simulink model "HW_InterleavedTotemBridgelessPFC_PR_V11_R2022a_AVE19"  (R2022a)
settings: Solver=FixedStepDiscrete  StartTime=0.0  StopTime=0.5  FixedStep=Ts_Power  RelTol=1e-3
InitFcn:
  | clc;
  | clear;
  | 
  | %%simulation paremeter
  | fsw = 130e3;%switch freq
  | Ts_Control = 1/fsw * 2;%control period
  | Ts_Power = 1 / fsw/128;%simulation step
  | Ts_Sample = 1 / fsw;%sample period
  | Tscon = Ts_Control;
  | %%system parameter
  | L = 250e-6;
  | L1 = L;
  | L2 = L;
  | C = 620e-6;
  | R = 75;
  | Uc_init = 390 ;%capacitor voltage init
  | v_ref = 390;
  | 
  | %%controller parameter
  | k_cp=-0.0235;
  | k_ci=-1.871e3;
  | 
  | k_vi = 1.7714;
  | k_vp = 0.0488;
undefined symbols (not defined in the file or in its folder): DiscIntNeverNeededParam
libraries: spsSeriesRLCBranchLib x3, slpidlib x2, spsCurrentMeasurementLib x2, spsVoltageMeasurementLib x2, spsACVoltageSourceLib x1, dsparch4 x1, spsPWMGenerator2LevelLib x1, spsStairGeneratorLib x1, spsTwoQuadrantDCDCConverterLib x1, spsUniversalBridgeLib x1, spspowerguiLib x1
settings Model: Creator=xg  LastModifiedBy=12586
settings SolverCC: AlgebraicLoopSolver=TrustRegion
settings DataIOCC: ReturnWorkspaceOutputs=off
settings DebuggingCC: ArithmeticOperatorsInVariantConditions=warning
settings SFSimCC: CustomCodeUndefinedFunction=UseInterfaceOnly

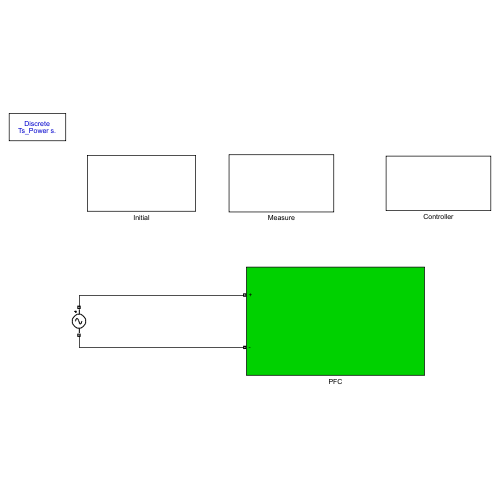
[thumbnail: Simulink's stored preview of the top-level diagram]
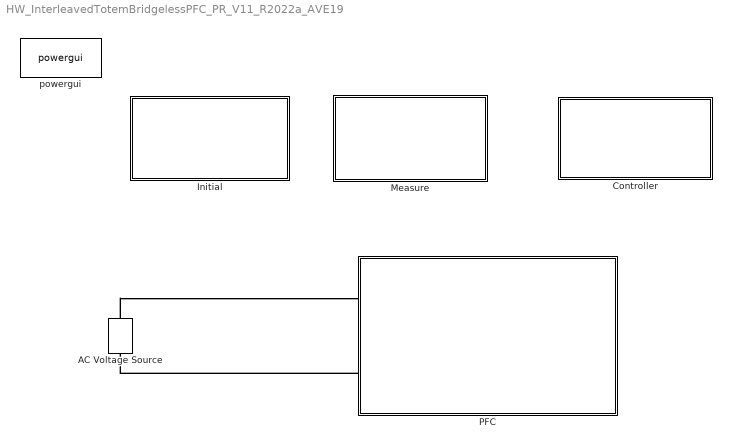
== system HW_InterleavedTotemBridgelessPFC_PR_V11_R2022a_AVE19 ==
  AC Voltage Source : spsACVoltageSourceLib/AC Voltage Source  Amplitude=220*sqrt(2)  Phase=0  Frequency=50  SampleTime=0  Measurements=None  BusType=swing  Pref=10e3  Qref=0  Qmin=-inf  Qmax=+inf
  Controller : Subsystem
  Initial : Subsystem
  Measure : Subsystem
  PFC : Subsystem
  powergui : spspowerguiLib/powergui  Priority=1  SimulationMode=Discrete  SampleTime=Ts_Power  frequency=60  Iterations=50  frequencyindice=0  Pbase=100e6  ErrMax=1e-4  UnitsV=kV  UnitsW=MW  buscounter=0  FunctionMessages=off  echomessages=off  EnableUseOfTLC=off  CurrentSourceSwitches=off  DisableSnubberDevices=off  DisableRonSwitches=off  DisableVfSwitches=off  DisplayEquations=off  AutomaticDiscreteSolvers=off  SolverType=Tustin/Backward Euler (TBE)  Interpol=off  ExternalGateDelay=off  methode=off  Ts=100  x0status=blocks  SPID=on  SwTol=0  HookPort=off  NonlinearTolerance=1e-4  nMaxIteration=100  ContinueOnMaxIteration=off  RestoreLinks=warning  ResistiveCurrentMeasurement=off  Frange=[0:2:500]  Ylog=off  Xlog=on  ShowGrid=off  save=off  variable=ZData  structure=logsout  ZoomFFT=on  StartTime=0.5  cycles=1  DisplayStyle=1  fundamental=50  FreqAxis=off  MaxFrequency=30000  frequencyindicesteady=1  RmsSteady=1  display=off
  connections:
  AC Voltage Source/RConn1 -- PFC/LConn1
  PFC/LConn2 -- AC Voltage Source/LConn1

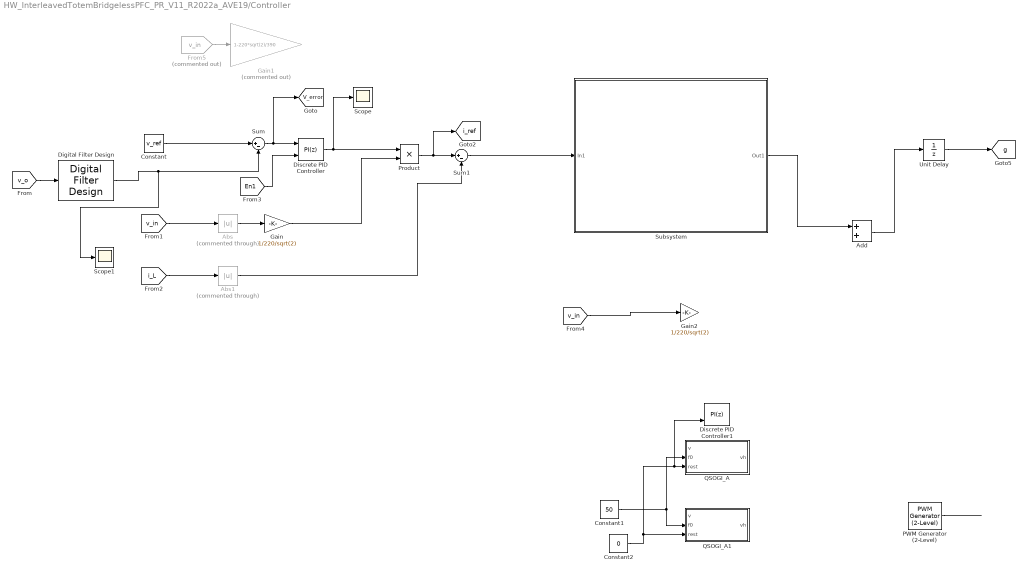
== system HW_InterleavedTotemBridgelessPFC_PR_V11_R2022a_AVE19/Controller ==
  Abs : Abs  Commented=through  SaturateOnIntegerOverflow=off
  Abs1 : Abs  Commented=through  SaturateOnIntegerOverflow=off
  Add : Sum
  Constant : Constant  Value=v_ref  SampleTime=Ts_Power
  Constant1 : Constant  Value=50  SampleTime=Ts_Power
  Constant2 : Constant  Value=0  SampleTime=Ts_Power
  Digital Filter Design : dsparch4/Digital Filter Design  mwdsp_browser_bugfix_var=off
  Discrete PID Controller : slpidlib/PID Controller  Controller=PI  Form=Parallel  TimeDomain=Discrete-time  UseExternalTs=off  SampleTime=Ts_Control  IntegratorMethod=Forward Euler  FilterMethod=Forward Euler  ControllerParametersSource=internal  P=k_vp  I=k_vi  UseKiTs=off  D=0  N=100  UseFilter=on  TunerSelectOption=Transfer Function Based (PID Tuner App)  InitialConditionSource=internal  InitialConditionForIntegrator=0  InitialConditionForFilter=0  DifferentiatorICPrevScaledInput=0  ExternalReset=level  TrackingMode=off  Kt=1  LimitOutput=off  SatLimitsSource=internal  UpperSaturationLimit=15  LowerSaturationLimit=0  LinearizeAsGain=off  AntiWindupMode=none  Kb=1  POutMin=[]  POutMax=[]  IOutMin=[]  IOutMax=[]  DOutMin=[]  DOutMax=[]  NOutMin=[]  NOutMax=[]  SumOutMin=[]  SumOutMax=[]  SaturationOutMin=[]  SaturationOutMax=[]  PParamMin=[]  PParamMax=[]  IParamMin=[]  IParamMax=[]  DParamMin=[]  DParamMax=[]  NParamMin=[]  NParamMax=[]  KbParamMin=[]  KbParamMax=[]  KtParamMin=[]  KtParamMax=[]  KbOutMin=[]  KbOutMax=[]  KtOutMin=[]  KtOutMax=[]  IntegratorOutMin=[]  IntegratorOutMax=[]  FilterOutMin=[]  FilterOutMax=[]  SumI1OutMin=[]  SumI1OutMax=[]  SumI2OutMin=[]  SumI2OutMax=[]  SumI3OutMin=[]  SumI3OutMax=[]  SumI4OutMin=[]  SumI4OutMax=[]  SumDOutMin=[]  SumDOutMax=[]  DifferentiatorOutMin=[]  DifferentiatorOutMax=[]  FilterDiffOutCoefMin=[]  FilterDiffOutCoefMax=[]  ReciprocalOutMin=[]  ReciprocalOutMax=[]  SumDenOutMin=[]  SumDenOutMax=[]  SumNumOutMin=[]  SumNumOutMax=[]  DivideOutMin=[]  DivideOutMax=[]  UdiffTsProdOutMin=[]  UdiffTsProdOutMax=[]  NTsProdOutMin=[]  NTsProdOutMax=[]  UintegralTsProdOutMin=[]  UintegralTsProdOutMax=[]  UngainTsProdOutMin=[]  UngainTsProdOutMax=[]  IntegratorContinuousStateAttributes=''  IntegratorStateMustResolveToSignalObject=off  IntegratorRTWStateStorageClass=Auto  FilterContinuousStateAttributes=''  FilterStateMustResolveToSignalObject=off  FilterRTWStateStorageClass=Auto  ParallelPVariant=InternalParameters  IdealPVariant=Disabled  IVariant=InternalParameters  DVariant=Disabled  IntegratorVariant=Discrete  SatVariant=Disabled  AWVariant=Passthrough  PCopyVariant=Disabled  TRVariant=Disabled  FdbkBlocksVariant=Forward  IdealPFdbkVariant=Disabled  SatFdbkVariant=Disabled  DerivativeFilterVariant=Disabled  NVariant=Disabled  NCopyVariant=Disabled_SignalSpec  FilterICVariant=Disabled  IntegratorICVariant=InternalICs  ExternalResetVariant=ExternalReset  TRSumVariant=Passthrough  SumFdbkVariant=Disabled  SumVariant=Sum_PI  TsampFilterVariant=InternalTs  TsampNgainVariant=Passthrough  TsampIntegralVariant=Passthrough  ExternalSaturationOutDataTypeStr=Inherit: Same as second input  aMode=0
  Discrete PID Controller1 : slpidlib/PID Controller  Controller=PI  Form=Parallel  TimeDomain=Discrete-time  UseExternalTs=off  SampleTime=Ts_Control  IntegratorMethod=Forward Euler  FilterMethod=Forward Euler  ControllerParametersSource=internal  P=k_cp  I=0  UseKiTs=off  D=0  N=100  UseFilter=on  TunerSelectOption=Transfer Function Based (PID Tuner App)  InitialConditionSource=internal  InitialConditionForIntegrator=0  InitialConditionForFilter=0  DifferentiatorICPrevScaledInput=0  ExternalReset=level  TrackingMode=off  Kt=1  LimitOutput=off  SatLimitsSource=internal  UpperSaturationLimit=1  LowerSaturationLimit=0  LinearizeAsGain=off  AntiWindupMode=none  Kb=1  POutMin=[]  POutMax=[]  IOutMin=[]  IOutMax=[]  DOutMin=[]  DOutMax=[]  NOutMin=[]  NOutMax=[]  SumOutMin=[]  SumOutMax=[]  SaturationOutMin=[]  SaturationOutMax=[]  PParamMin=[]  PParamMax=[]  IParamMin=[]  IParamMax=[]  DParamMin=[]  DParamMax=[]  NParamMin=[]  NParamMax=[]  KbParamMin=[]  KbParamMax=[]  KtParamMin=[]  KtParamMax=[]  KbOutMin=[]  KbOutMax=[]  KtOutMin=[]  KtOutMax=[]  IntegratorOutMin=[]  IntegratorOutMax=[]  FilterOutMin=[]  FilterOutMax=[]  SumI1OutMin=[]  SumI1OutMax=[]  SumI2OutMin=[]  SumI2OutMax=[]  SumI3OutMin=[]  SumI3OutMax=[]  SumI4OutMin=[]  SumI4OutMax=[]  SumDOutMin=[]  SumDOutMax=[]  DifferentiatorOutMin=[]  DifferentiatorOutMax=[]  FilterDiffOutCoefMin=[]  FilterDiffOutCoefMax=[]  ReciprocalOutMin=[]  ReciprocalOutMax=[]  SumDenOutMin=[]  SumDenOutMax=[]  SumNumOutMin=[]  SumNumOutMax=[]  DivideOutMin=[]  DivideOutMax=[]  UdiffTsProdOutMin=[]  UdiffTsProdOutMax=[]  NTsProdOutMin=[]  NTsProdOutMax=[]  UintegralTsProdOutMin=[]  UintegralTsProdOutMax=[]  UngainTsProdOutMin=[]  UngainTsProdOutMax=[]  IntegratorContinuousStateAttributes=''  IntegratorStateMustResolveToSignalObject=off  IntegratorRTWStateStorageClass=Auto  FilterContinuousStateAttributes=''  FilterStateMustResolveToSignalObject=off  FilterRTWStateStorageClass=Auto  ParallelPVariant=InternalParameters  IdealPVariant=Disabled  IVariant=InternalParameters  DVariant=Disabled  IntegratorVariant=Discrete  SatVariant=Disabled  AWVariant=Passthrough  PCopyVariant=Disabled  TRVariant=Disabled  FdbkBlocksVariant=Forward  IdealPFdbkVariant=Disabled  SatFdbkVariant=Disabled  DerivativeFilterVariant=Disabled  NVariant=Disabled  NCopyVariant=Disabled_SignalSpec  FilterICVariant=Disabled  IntegratorICVariant=InternalICs  ExternalResetVariant=ExternalReset  TRSumVariant=Passthrough  SumFdbkVariant=Disabled  SumVariant=Sum_PI  TsampFilterVariant=InternalTs  TsampNgainVariant=Passthrough  TsampIntegralVariant=Passthrough  ExternalSaturationOutDataTypeStr=Inherit: Same as second input  aMode=0
  From5 : From  Commented=on  GotoTag=v_in  TagVisibility=global
  Gain : Gain  Gain=1/220/sqrt(2)
  Gain1 : Gain  Commented=on  Gain=1-220*sqrt(2)/390
  Gain2 : Gain  Gain=1/220/sqrt(2)
  PWM Generator (2-Level) : spsPWMGenerator2LevelLib/PWM Generator (2-Level)  ModulatorType=Single-phase half-bridge (2 pulses)  ModulatorMode=Unsynchronized  Fc=130e3  Pc=0  nF=27  MinMax="[ 0  1 ]"  SamplingTechnique=Symmetrical regular (single edge)  ModulatingSignals=off  m=0.8  Freq=60  Phase=0  Ts=Ts_Power  ShowCarrierOutport=off
  Product : Product
  QSOGI_A : Subsystem  mask{h=1, KIh=-86, wc=0.002, phch=0.0036, Ts=Ts_Control}
      mask prompts: h "Selected harmonic orders"; KIh "Integral gain of QSOGI"; wc "Inversion of maximum gain"; phch "Phase compensation angle"; Ts "Sampling Period"
      mask Display: disp('QSOGIh(z)')
  QSOGI_A1 : Subsystem  mask{h=3, KIh=200, wc=0.002, phch=1.5*Ts_Control*2*pi*150, Ts=Ts_Control}
      mask prompts: h "Selected harmonic orders"; KIh "Integral gain of QSOGI"; wc "Inversion of maximum gain"; phch "Phase compensation angle"; Ts "Sampling Period"
      mask Display: disp('QSOGIh(z)')
  Scope : Scope
  Scope1 : Scope
  Subsystem : Subsystem
  Sum : Sum  Inputs=|+-
  Sum1 : Sum  Inputs=|+-
  Unit Delay : UnitDelay  SampleTime=Ts_Control  HasFrameUpgradeWarning=on
  tag scope: V_error=global, g=global, i_ref=global
  wires:
  Constant2/1 -> Discrete PID Controller1/2, QSOGI_A/3(rest), QSOGI_A1/3(rest)
  [En1] -> Discrete PID Controller/2
  [v_o] -> Digital Filter Design/1
  Constant/1 -> Sum/1
  Sum/1 -> Discrete PID Controller/1, [V_error]
  [v_in] -> Abs/1
  [i_L] -> Abs1/1
  Abs/1 -> Gain/1
  Abs1/1 -> Sum1/2
  Product/1 -> [i_ref], Sum1/1
  Gain/1 -> Product/2
  Discrete PID Controller/1 -> Scope/1, Product/1
  From5/1 -> Gain1/1
  Constant1/1 -> QSOGI_A/2(f0), QSOGI_A1/2(f0)
  ? -> PWM Generator (2-Level)/1
  PWM Generator (2-Level)/1 -> ?
  Unit Delay/1 -> [g]
  Add/1 -> Unit Delay/1
  Sum1/1 -> Subsystem/1(In1)
  Subsystem/1(Out1) -> Add/1
  [v_in] -> Gain2/1
  Digital Filter Design/1 -> Scope1/1, Sum/2

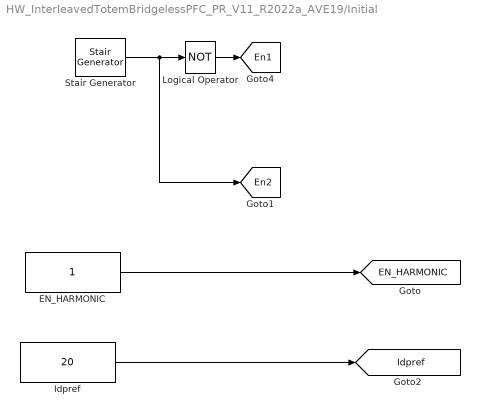
== system HW_InterleavedTotemBridgelessPFC_PR_V11_R2022a_AVE19/Initial ==
  EN_HARMONIC : Constant  SampleTime=Ts_Control
  Idpref : Constant  Value=20  SampleTime=Ts_Control
  Logical Operator : Logic  Operator=NOT  AllPortsSameDT=off  OutDataTypeStr=boolean
  Stair Generator : spsStairGeneratorLib/Stair Generator  t=[0, 0.01]  e=[0, 1]  Ts=0
  tag scope: EN_HARMONIC=global, En1=global, En2=global, Idpref=global
  wires:
  Stair Generator/1 -> [En2], Logical Operator/1
  Logical Operator/1 -> [En1]
  EN_HARMONIC/1 -> [EN_HARMONIC]
  Idpref/1 -> [Idpref]

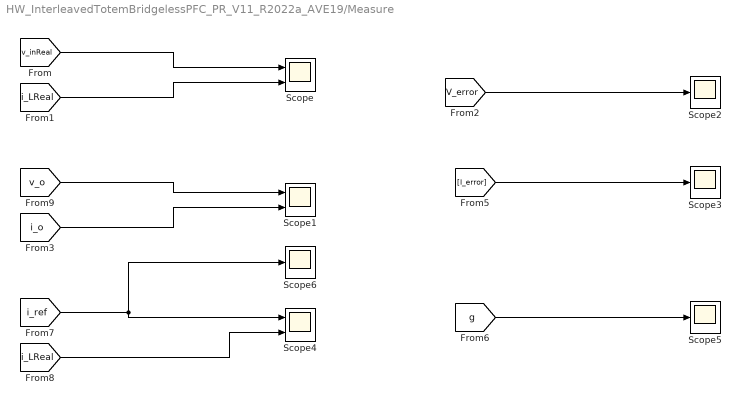
== system HW_InterleavedTotemBridgelessPFC_PR_V11_R2022a_AVE19/Measure ==
  Scope : Scope  NumInputPorts=2
  Scope1 : Scope  NumInputPorts=2
  Scope{2..3,5..6} (4 alike) : Scope
  Scope4 : Scope  NumInputPorts=2
  wires:
  [v_inReal] -> Scope/1
  [i_LReal] -> Scope/2
  [V_error] -> Scope2/1
  [I_error] -> Scope3/1
  [i_ref] -> Scope6/1, Scope4/1
  [g] -> Scope5/1
  [i_LReal] -> Scope4/2
  [v_o] -> Scope1/1
  [i_o] -> Scope1/2

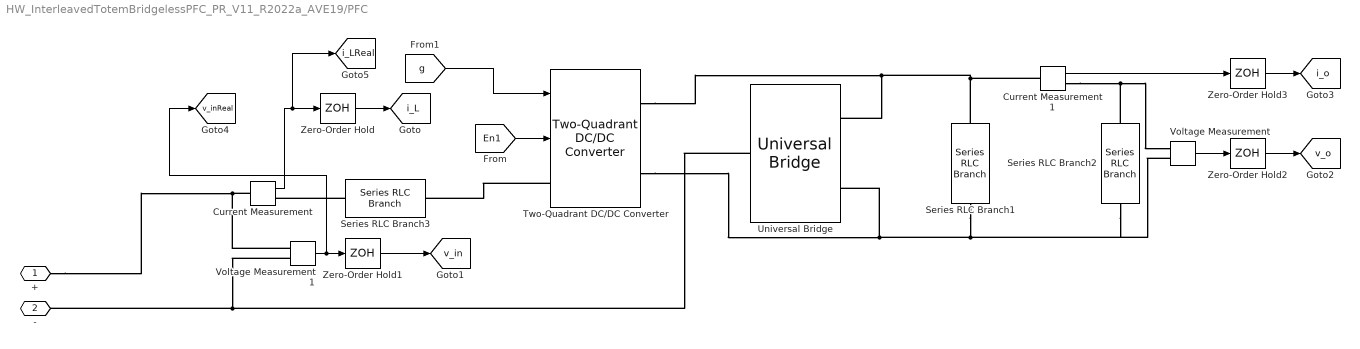
== system HW_InterleavedTotemBridgelessPFC_PR_V11_R2022a_AVE19/PFC ==
  Current Measurement : spsCurrentMeasurementLib/Current Measurement  PhasorSimulation=off  OutputType=Complex  PSBequivalent=0
  Current Measurement1 : spsCurrentMeasurementLib/Current Measurement  PhasorSimulation=off  OutputType=Complex  PSBequivalent=0
  Series RLC Branch1 : spsSeriesRLCBranchLib/Series RLC Branch  LConnTagsString=__new0  RConnTagsString=__new0  BranchType=C  Resistance=1  Inductance=1e-3  SetiL0=off  InitialCurrent=0  Capacitance=C  Setx0=on  InitialVoltage=Uc_init  Measurements=None
  Series RLC Branch2 : spsSeriesRLCBranchLib/Series RLC Branch  LConnTagsString=__new0  RConnTagsString=__new0  BranchType=R  Resistance=R  Inductance=1e-3  SetiL0=off  InitialCurrent=0  Capacitance=1e-6  Setx0=off  InitialVoltage=0  Measurements=None
  Series RLC Branch3 : spsSeriesRLCBranchLib/Series RLC Branch  LConnTagsString=__new0  RConnTagsString=__new0  BranchType=L  Resistance=75  Inductance=L  SetiL0=off  InitialCurrent=0  Capacitance=1e-6  Setx0=off  InitialVoltage=0  Measurements=None
  Two-Quadrant DC/DC Converter : spsTwoQuadrantDCDCConverterLib/Two-Quadrant DC//DC Converter  ModelType=Average model (D-controlled)  Ron=1e-3  Rs=1e6  Cs=inf  Vforward=[0,0]  Ron_Diode=1e-6  Rs_Diode=1e6  Cs_Diode=inf  Vf_Diode=1e-6  Rs_CurrentSource=inf  Ron_ACsource=1e-3
      settings: SourceProductBaseCode=PS
  Universal Bridge : spsUniversalBridgeLib/Universal Bridge  Arms=1  SnubberResistance=1e5  SnubberCapacitance=inf  Device=Diodes  Ron=1e-3  Lon=0  ForwardVoltages="[  0  0  ]"  ForwardVoltage=0  GTOparameters=[ 10e-6 , 20e-6 ]  IGBTparameters=[ 1e-6 , 2e-6 ]  Measurements=None  Measurements_2=None  converterType=Rectifier
  Voltage Measurement : spsVoltageMeasurementLib/Voltage Measurement  PhasorSimulation=off  OutputType=Complex  PSBequivalent=0
  Voltage Measurement1 : spsVoltageMeasurementLib/Voltage Measurement  PhasorSimulation=off  OutputType=Complex  PSBequivalent=0
  Zero-Order Hold{,1..3} (4 alike) : ZeroOrderHold  SampleTime=Ts_Sample
  + : PMIOPort  Side=Left
  - : PMIOPort  Port=2  Side=Left
  tag scope: i_L=global, i_LReal=global, i_o=global, v_in=global, v_inReal=global, v_o=global
  wires:
  Voltage Measurement1/1 -> [v_inReal], Zero-Order Hold1/1
  Zero-Order Hold2/1 -> [v_o]
  Zero-Order Hold/1 -> [i_L]
  Current Measurement/1 -> [i_LReal], Zero-Order Hold/1
  Voltage Measurement/1 -> Zero-Order Hold2/1
  [g] -> Two-Quadrant DC/DC Converter/1
  Current Measurement1/1 -> Zero-Order Hold3/1
  Zero-Order Hold1/1 -> [v_in]
  Zero-Order Hold3/1 -> [i_o]
  [En1] -> Two-Quadrant DC/DC Converter/2
  connections:
  Current Measurement/LConn1 -- +/RConn1 -- Voltage Measurement1/LConn1
  Series RLC Branch2/RConn1 -- Voltage Measurement/LConn2 -- Series RLC Branch1/RConn1 -- Two-Quadrant DC/DC Converter/RConn2 -- Universal Bridge/RConn2
  Voltage Measurement1/LConn2 -- Universal Bridge/LConn1 -- -/RConn1
  Series RLC Branch3/LConn1 -- Current Measurement/RConn1
  Series RLC Branch2/LConn1 -- Current Measurement1/RConn1 -- Voltage Measurement/LConn1
  Current Measurement1/LConn1 -- Two-Quadrant DC/DC Converter/RConn1 -- Universal Bridge/RConn1 -- Series RLC Branch1/LConn1
  Two-Quadrant DC/DC Converter/LConn1 -- Series RLC Branch3/RConn1

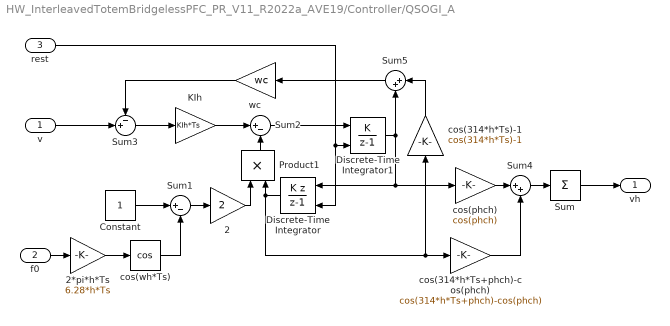
== system HW_InterleavedTotemBridgelessPFC_PR_V11_R2022a_AVE19/Controller/QSOGI_A ==
  v : Inport
  f0 : Inport  Port=2
  rest : Inport  Port=3
  2 : Gain  Gain=2
  2*pi*h*Ts : Gain  Gain=6.28*h*Ts
  Constant : Constant  SampleTime=Tscon
  Discrete-Time Integrator : DiscreteIntegrator  IntegratorMethod=Accumulation: Backward Euler  ExternalReset=level  SampleTime=-1  ICPrevOutput=DiscIntNeverNeededParam  ICPrevScaledInput=DiscIntNeverNeededParam
  Discrete-Time Integrator1 : DiscreteIntegrator  IntegratorMethod=Accumulation: Forward Euler  ExternalReset=level  SampleTime=-1  ICPrevOutput=DiscIntNeverNeededParam  ICPrevScaledInput=DiscIntNeverNeededParam
  KIh : Gain  Gain=KIh*Ts
  Product1 : Product
  Sum : Sum  Inputs=+
  Sum1 : Sum  Inputs=|+-
  Sum2 : Sum  Inputs=|+-
  Sum3 : Sum  Inputs=-+|
  Sum4 : Sum  Inputs=|++
  Sum5 : Sum  Inputs=|++
  cos(314*h*Ts)-1 : Gain  Gain=cos(314*h*Ts)-1
  cos(314*h*Ts+phch)-cos(phch) : Gain  Gain=cos(314*h*Ts+phch)-cos(phch)
  cos(phch) : Gain  Gain=cos(phch)
  cos(wh*Ts) : Trigonometry  Operator=cos
  wc : Gain  Gain=wc
  vh : Outport  VectorParamsAs1DForOutWhenUnconnected=off
  wires:
  rest/1 -> Discrete-Time Integrator1/2, Discrete-Time Integrator/2
  Product1/1 -> Sum2/2
  Sum2/1 -> Discrete-Time Integrator1/1
  v/1 -> Sum3/2
  KIh/1 -> Sum2/1
  f0/1 -> 2*pi*h*Ts/1
  Discrete-Time Integrator1/1 -> Discrete-Time Integrator/1, cos(phch)/1, Sum5/2
  Discrete-Time Integrator/1 -> cos(314*h*Ts)-1/1, cos(314*h*Ts+phch)-cos(phch)/1, Product1/2
  Sum4/1 -> Sum/1
  2*pi*h*Ts/1 -> cos(wh*Ts)/1
  cos(wh*Ts)/1 -> Sum1/2
  Constant/1 -> Sum1/1
  Sum1/1 -> 2/1
  2/1 -> Product1/1
  cos(phch)/1 -> Sum4/1
  cos(314*h*Ts+phch)-cos(phch)/1 -> Sum4/2
  Sum/1 -> vh/1
  wc/1 -> Sum3/1
  Sum3/1 -> KIh/1
  Sum5/1 -> wc/1
  cos(314*h*Ts)-1/1 -> Sum5/1

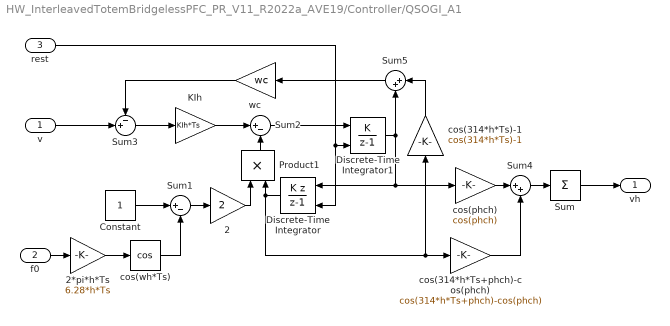
== system HW_InterleavedTotemBridgelessPFC_PR_V11_R2022a_AVE19/Controller/QSOGI_A1 ==
  v : Inport
  f0 : Inport  Port=2
  rest : Inport  Port=3
  2 : Gain  Gain=2
  2*pi*h*Ts : Gain  Gain=6.28*h*Ts
  Constant : Constant  SampleTime=Tscon
  Discrete-Time Integrator : DiscreteIntegrator  IntegratorMethod=Accumulation: Backward Euler  ExternalReset=level  SampleTime=-1  ICPrevOutput=DiscIntNeverNeededParam  ICPrevScaledInput=DiscIntNeverNeededParam
  Discrete-Time Integrator1 : DiscreteIntegrator  IntegratorMethod=Accumulation: Forward Euler  ExternalReset=level  SampleTime=-1  ICPrevOutput=DiscIntNeverNeededParam  ICPrevScaledInput=DiscIntNeverNeededParam
  KIh : Gain  Gain=KIh*Ts
  Product1 : Product
  Sum : Sum  Inputs=+
  Sum1 : Sum  Inputs=|+-
  Sum2 : Sum  Inputs=|+-
  Sum3 : Sum  Inputs=-+|
  Sum4 : Sum  Inputs=|++
  Sum5 : Sum  Inputs=|++
  cos(314*h*Ts)-1 : Gain  Gain=cos(314*h*Ts)-1
  cos(314*h*Ts+phch)-cos(phch) : Gain  Gain=cos(314*h*Ts+phch)-cos(phch)
  cos(phch) : Gain  Gain=cos(phch)
  cos(wh*Ts) : Trigonometry  Operator=cos
  wc : Gain  Gain=wc
  vh : Outport  VectorParamsAs1DForOutWhenUnconnected=off
  wires:
  cos(314*h*Ts)-1/1 -> Sum5/1
  Sum5/1 -> wc/1
  Sum3/1 -> KIh/1
  wc/1 -> Sum3/1
  Sum/1 -> vh/1
  cos(314*h*Ts+phch)-cos(phch)/1 -> Sum4/2
  cos(phch)/1 -> Sum4/1
  2/1 -> Product1/1
  Sum1/1 -> 2/1
  Constant/1 -> Sum1/1
  cos(wh*Ts)/1 -> Sum1/2
  2*pi*h*Ts/1 -> cos(wh*Ts)/1
  Sum4/1 -> Sum/1
  Discrete-Time Integrator/1 -> Product1/2, cos(314*h*Ts+phch)-cos(phch)/1, cos(314*h*Ts)-1/1
  Discrete-Time Integrator1/1 -> Sum5/2, cos(phch)/1, Discrete-Time Integrator/1
  f0/1 -> 2*pi*h*Ts/1
  KIh/1 -> Sum2/1
  v/1 -> Sum3/2
  Sum2/1 -> Discrete-Time Integrator1/1
  Product1/1 -> Sum2/2
  rest/1 -> Discrete-Time Integrator/2, Discrete-Time Integrator1/2

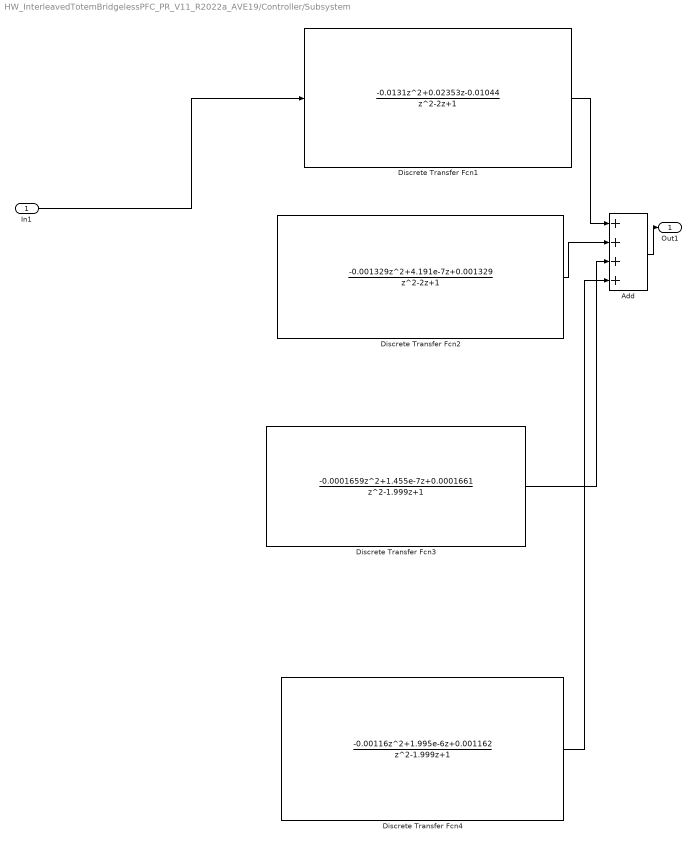
== system HW_InterleavedTotemBridgelessPFC_PR_V11_R2022a_AVE19/Controller/Subsystem ==
  In1 : Inport
  Add : Sum  Inputs=++++
  Discrete Transfer Fcn1 : DiscreteTransferFcn  Numerator=[-0.0131,0.02353,-0.01044]  Denominator=[1 -2 1]  SampleTime=Ts_Control
  Discrete Transfer Fcn2 : DiscreteTransferFcn  Numerator=[-0.001329,4.191e-7,0.001329]  Denominator=[1 -2 1]  SampleTime=Ts_Control
  Discrete Transfer Fcn3 : DiscreteTransferFcn  Numerator=[-0.0001659,1.455e-7,0.0001661]  Denominator=[1 -1.999 1]  SampleTime=Ts_Control
  Discrete Transfer Fcn4 : DiscreteTransferFcn  Numerator=[-0.00116,1.995e-6,0.001162]  Denominator=[1 -1.999 1]  SampleTime=Ts_Control
  Out1 : Outport
  wires:
  Discrete Transfer Fcn1/1 -> Add/1
  Discrete Transfer Fcn2/1 -> Add/2
  Add/1 -> Out1/1
  Discrete Transfer Fcn3/1 -> Add/3
  Discrete Transfer Fcn4/1 -> Add/4
  In1/1 -> Discrete Transfer Fcn1/1
